simulink model "Programmable_Source"  (R2014a)
settings: Solver=ode45  StartTime=0.0  StopTime=10.0  RelTol=1e-3
undefined symbols (not defined in the file): sigbuilder_block, Ts
settings Model: Creator=User  LastModifiedBy=User

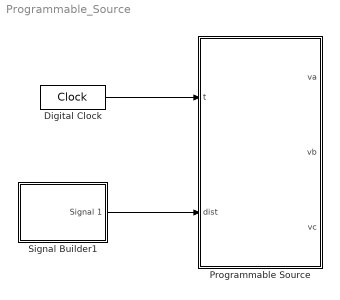
== system Programmable_Source ==
  Digital Clock : DigitalClock  SampleTime=Ts
  Programmable Source : MATLAB Function  TreatAsAtomicUnit=on
  Signal Builder1 : Subsystem  Tag=STV Subsys  LoadFcn=sigbuilder_block('load');  StartFcn=sigbuilder_block('start');  StopFcn=sigbuilder_block('stop');  ClipboardFcn=sigbuilder_block('clipboard');  mask(Sigbuilder block){}
      mask help: Simulink:masks:SigbuilderBlock_MD
      mask init:
      | if ~strcmp(get_param(bdroot(gcbh),'SimulationStatus'),'stopped') tuvar = sigbuilder_block('maskInit'); end
      settings: CopyFcn=sigbuilder_block('copy');  DeleteFcn=sigbuilder_block('delete');  ModelCloseFcn=sigbuilder_block('modelClose');  PreSaveFcn=sigbuilder_block('preSave');  PauseFcn=sigbuilder_block('pause');  ContinueFcn=sigbuilder_block('continue');  NameChangeFcn=sigbuilder_block('namechange');  OpenFcn=sigbuilder_block('open',[306 85.5 550.5 394.5 ]);  CloseFcn=sigbuilder_block('close');
      mask Display: plot(0, 0, 100, 100,[2, 2, 32, 32, 2], [68, 8, 8, 68, 68],[32, 2], [38, 38], [32, 19, 2],[53, 60, 44], [32, 17, 17, 2],[16, 16, 31, 31]);txt = getActiveGroup(gcbh);text(2, 100, txt,'verticalAlignment', 'top');
  wires:
  Digital Clock/1 -> Programmable Source/1(t)
  Signal Builder1/1(Signal 1) -> Programmable Source/2(dist)

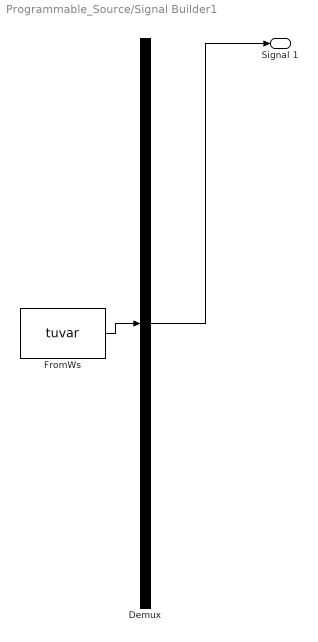
== system Programmable_Source/Signal Builder1 ==
  Demux : Demux  Tag=STV Demux  Outputs=1
  FromWs : FromWorkspace  Tag=STV FromWs  VariableName=tuvar  SampleTime=0
      SigBuilderData=|
      | common.afterFinalStr = 'Extrapolate'
      | common.sampleTime = 0
      | dataSet.timeRange = [0 3]
      | dataSet.name = 'Group 1'
      | sbobj.Groups.Name = 'Group 1'
      | sbobj.Groups.Signals.Name = 'Signal 1'
      | sbobj.Groups.Signals.XData = [0 0.6 0.6 0.8 0.8 1 1 1.2 1.2 1.4 1.4 1.6 1.6 1.8 1.8 2 2 2.2 2.2 2.4 2.4 2.6 2.6 3]
      | sbobj.Groups.Signals.YData = [1 1 2 2 3 3 4 4 5 5 6 6 7 7 8 8 9 9 10 10 11 11 11.85 11.85]
      | sbobj.Groups.TimeRange = [0 3]
  Signal 1 : Outport  Tag=STV Outport
  wires:
  FromWs/1 -> Demux/1
  Demux/1 -> Signal 1/1

== matlab function Programmable_Source/Programmable Source ==
  data: t input; va output; vb output; vc output; dist input
function [va, vb, vc] = fcn(t,dist)
%#codegen
% phase angle difference between a and b
f = 50;
w1 = 2*pi*f;  % For variable frequency operation
 w = w1;     % Use it for variable freq operation
%w = 2*pi*50; % For constant frequency operation
Vm = 325; % Peak of source voltage

%
if dist == 1         % Normal operation
    va1 = Vm*sin(w*t);
    vb1 = Vm*sin((w*t)-(2*pi/3));
    vc1 = Vm*sin((w*t)+(2*pi/3));
    
    va5 = 0;    vb5 = 0;      vc5 = 0;
    va7 = 0;    vb7 = 0;      vc7 = 0;
    va11 = 0;   vb11 = 0;     vc11 = 0;
    va13 = 0;   vb13 = 0;     vc13 = 0;
    
    
    
elseif dist == 2       % Fundamental Balanced sag of 0.5 pu
    va1 = 0.5*Vm*sin(w*t);
    vb1 = 0.5*Vm*sin((w*t)-(2*pi/3));
    vc1 = 0.5*Vm*sin((w*t)+(2*pi/3));
    
    va5 = 0;    vb5 = 0;      vc5 = 0;
    va7 = 0;    vb7 = 0;      vc7 = 0;
    va11 = 0;   vb11 = 0;     vc11 = 0;
    va13 = 0;   vb13 = 0;     vc13 = 0;
    
    
    
elseif dist == 3         % Fundamental Unbalanced sag Va = 0.5 pu and others at 1 pu
    va1 = 0.5*Vm*sin(w*t);
    vb1 = Vm*sin((w*t)-(2*pi/3));
    vc1 = Vm*sin((w*t)+(2*pi/3));
    
    va5 = 0;    vb5 = 0;      vc5 = 0;
    va7 = 0;    vb7 = 0;      vc7 = 0;
    va11 = 0;   vb11 = 0;     vc11 = 0;
    va13 = 0;   vb13 = 0;     vc13 = 0;
    
    
    
elseif dist == 4                     % Fundamental Balanced swell of 1.2 pu
    va1 = 1.2*Vm*sin(w*t);
    vb1 = 1.2*Vm*sin((w*t)-(2*pi/3));
    vc1 = 1.2*Vm*sin((w*t)+(2*pi/3));
    
    va5 = 0;    vb5 = 0;      vc5 = 0;
    va7 = 0;    vb7 = 0;      vc7 = 0;
    va11 = 0;   vb11 = 0;     vc11 = 0;
    va13 = 0;   vb13 = 0;     vc13 = 0;
    
    
elseif dist == 5       % Fundamental unbalanced swell Va = 1.2 pu and others at 1pu
    va1 = 1.2*Vm*sin(w*t);
    vb1 = Vm*sin((w*t)-(2*pi/3));
    vc1 = Vm*sin((w*t)+(2*pi/3));
    
    va5 = 0;    vb5 = 0;      vc5 = 0;
    va7 = 0;    vb7 = 0;      vc7 = 0;
    va11 = 0;   vb11 = 0;     vc11 = 0;
    va13 = 0;   vb13 = 0;     vc13 = 0;
    
    
elseif dist == 6      % Distorted Grid
    va1 = Vm*sin(w*t);
    vb1 = Vm*sin((w*t)-(2*pi/3));
    vc1 = Vm*sin((w*t)+(2*pi/3));
    
    va5 = 0.2*Vm*sin(5*w*t)/4;
    vb5 = 0.2*Vm*sin((5*w*t)-(5*2*pi/3))/4;
    vc5 = 0.2*Vm*sin((5*w*t)+(5*2*pi/3))/4;
    
    va7 = (Vm*sin(7*w*t))/(7*4);
    vb7 = (Vm*sin((7*w*t)-(7*2*pi/3)))/(7*4);
    vc7 = (Vm*sin((7*w*t)+(7*2*pi/3)))/(7*4);
    
    va11 = (Vm*sin(11*w*t))/(11*1);
    vb11 = (Vm*sin((11*w*t)-(11*2*pi/3)))/(11*1);
    vc11 = (Vm*sin((11*w*t)+(11*2*pi/3)))/(11*1);
    
    va13 = (Vm*sin(13*w*t))/(13*1);
    vb13 = (Vm*sin((13*w*t)-(13*2*pi/3)))/(13*1);
    vc13 = (Vm*sin((13*w*t)+(13*2*pi/3)))/(13*1);
    
   
elseif dist == 7      % Distorted Grid with balanced sag of 0.5 pu
    va1 = 0.5*Vm*sin(w*t);
    vb1 = 0.5*Vm*sin((w*t)-(2*pi/3));
    vc1 = 0.5*Vm*sin((w*t)+(2*pi/3));
    
    va5 = 0.2*0.5*Vm*sin(5*w*t)/4;
    vb5 = 0.2*0.5*Vm*sin((5*w*t)-(5*2*pi/3))/4;
    vc5 = 0.2*0.5*Vm*sin((5*w*t)+(5*2*pi/3))/4;
    
    va7 = (0.5*Vm*sin(7*w*t))/(7*4);
    vb7 = (0.5*Vm*sin((7*w*t)-(7*2*pi/3)))/(7*4);
    vc7 = (0.5*Vm*sin((7*w*t)+(7*2*pi/3)))/(7*4);
    
    va11 = (0.5*Vm*sin(11*w*t))/(11*1);
    vb11 = (0.5*Vm*sin((11*w*t)-(11*2*pi/3)))/(11*1);
    vc11 = (0.5*Vm*sin((11*w*t)+(11*2*pi/3)))/(11*1);
    
    va13 = (0.5*Vm*sin(13*w*t))/(13*1);
    vb13 = (0.5*Vm*sin((13*w*t)-(13*2*pi/3)))/(13*1);
    vc13 = (0.5*Vm*sin((13*w*t)+(13*2*pi/3)))/(13*1);
    
    
elseif dist == 8      % Distorted Grid with unbalanced sag Va = 0.5 pu and other at 1 pu
    va1 = 0.5*Vm*sin(w*t);
    vb1 = Vm*sin((w*t)-(2*pi/3));
    vc1 = Vm*sin((w*t)+(2*pi/3));
    
    va5 = 0.2*0.5*Vm*sin(5*w*t)/4;
    vb5 = 0.2*Vm*sin((5*w*t)-(5*2*pi/3))/4;
    vc5 = 0.2*Vm*sin((5*w*t)+(5*2*pi/3))/4;
    
    va7 = (0.5*Vm*sin(7*w*t))/(7*4);
    vb7 = (Vm*sin((7*w*t)-(7*2*pi/3)))/(7*4);
    vc7 = (Vm*sin((7*w*t)+(7*2*pi/3)))/(7*4);
    
    va11 = (0.5*Vm*sin(11*w*t))/(11*1);
    vb11 = (Vm*sin((11*w*t)-(11*2*pi/3)))/(11*1);
    vc11 = (Vm*sin((11*w*t)+(11*2*pi/3)))/(11*1);
    
    va13 = (0.5*Vm*sin(13*w*t))/(13*1);
    vb13 = (Vm*sin((13*w*t)-(13*2*pi/3)))/(13*1);
    vc13 = (Vm*sin((13*w*t)+(13*2*pi/3)))/(13*1);
    
    
elseif dist == 9      % Distorted Grid with balanced swell of 1.2 pu.
    va1 = 1.2*Vm*sin(w*t);
    vb1 = 1.2*Vm*sin((w*t)-(2*pi/3));
    vc1 = 1.2*Vm*sin((w*t)+(2*pi/3));
    
    va5 = 0.2*1.2*Vm*sin(5*w*t)/4;
    vb5 = 0.2*1.2*Vm*sin((5*w*t)-(5*2*pi/3))/4;
    vc5 = 0.2*1.2*Vm*sin((5*w*t)+(5*2*pi/3))/4;
    
    va7 = (1.2*Vm*sin(7*w*t))/(7*4);
    vb7 = (1.2*Vm*sin((7*w*t)-(7*2*pi/3)))/(7*4);
    vc7 = (1.2*Vm*sin((7*w*t)+(7*2*pi/3)))/(7*4);
    
    va11 = (1.2*Vm*sin(11*w*t))/(11*1);
    vb11 = (1.2*Vm*sin((11*w*t)-(11*2*pi/3)))/(11*1);
    vc11 = (1.2*Vm*sin((11*w*t)+(11*2*pi/3)))/(11*1);
    
    va13 = (1.2*Vm*sin(13*w*t))/(13*1);
    vb13 = (1.2*Vm*sin((13*w*t)-(13*2*pi/3)))/(13*1);
    vc13 = (1.2*Vm*sin((13*w*t)+(13*2*pi/3)))/(13*1);
    
    
elseif dist == 10      % Distorted Grid with unbalanced swell Va = 1.2 pu and others at 1 pu.
    va1 = 1.2*Vm*sin(w*t);
    vb1 = Vm*sin((w*t)-(2*pi/3));
    vc1 = Vm*sin((w*t)+(2*pi/3));
    
    va5 = 0.2*1.2*Vm*sin(5*w*t)/4;
    vb5 = 0.2*Vm*sin((5*w*t)-(5*2*pi/3))/4;
    vc5 = 0.2*Vm*sin((5*w*t)+(5*2*pi/3))/4;
    
    va7 = (1.2*Vm*sin(7*w*t))/(7*4);
    vb7 = (Vm*sin((7*w*t)-(7*2*pi/3)))/(7*4);
    vc7 = (Vm*sin((7*w*t)+(7*2*pi/3)))/(7*4);
    
    va11 = (1.2*Vm*sin(11*w*t))/(11*1);
    vb11 = (Vm*sin((11*w*t)-(11*2*pi/3)))/(11*1);
    vc11 = (Vm*sin((11*w*t)+(11*2*pi/3)))/(11*1);
    
    va13 = (1.2*Vm*sin(13*w*t))/(13*1);
    vb13 = (Vm*sin((13*w*t)-(13*2*pi/3)))/(13*1);
    vc13 = (Vm*sin((13*w*t)+(13*2*pi/3)))/(13*1);
    
    
elseif dist == 11         % Shunt shorting case
    va1 = 1.8*Vm*sin(w*t);
    vb1 = 1.8*Vm*sin((w*t)-(2*pi/3));
    vc1 = 1.8*Vm*sin((w*t)+(2*pi/3));
    
    va5 = 0.2*1.8*Vm*sin(5*w*t)/4;
    vb5 = 0.2*1.8*Vm*sin((5*w*t)-(5*2*pi/3))/4;
    vc5 = 0.2*1.8*Vm*sin((5*w*t)+(5*2*pi/3))/4;
    
    va7 = (1.8*Vm*sin(7*w*t))/(7*4);
    vb7 = (1.8*Vm*sin((7*w*t)-(7*2*pi/3)))/(7*4);
    vc7 = (1.8*Vm*sin((7*w*t)+(7*2*pi/3)))/(7*4);
    
    va11 = (1.8*Vm*sin(11*w*t))/(11*1);
    vb11 = (1.8*Vm*sin((11*w*t)-(11*2*pi/3)))/(11*1);
    vc11 = (1.8*Vm*sin((11*w*t)+(11*2*pi/3)))/(11*1);
    
    va13 = (1.8*Vm*sin(13*w*t))/(13*1);
    vb13 = (1.8*Vm*sin((13*w*t)-(13*2*pi/3)))/(13*1);
    vc13 = (1.8*Vm*sin((13*w*t)+(13*2*pi/3)))/(13*1);
    
    
else
    va1 = 1*Vm*sin(w*t);
    vb1 = 1*Vm*sin((w*t)-(2*pi/3));
    vc1 = 1*Vm*sin((w*t)+(2*pi/3));
    
    va5 = 0;    vb5 = 0;      vc5 = 0;
    va7 = 0;    vb7 = 0;      vc7 = 0;
    va11 = 0;   vb11 = 0;     vc11 = 0;
    va13 = 0;   vb13 = 0;     vc13 = 0;
    
    
end
%}

va = va1 + va5 + va7 + va11 + va13;
vb = vb1 + vb5 + vb7 + vb11 + vb13;
vc = vc1 + vc5 + vc7 + vc11 + vc13;
